simulink model "D_TrigSubsysSin"  (R2019b)
settings: Solver=FixedStepAuto  StartTime=0.0  StopTime=10  FixedStep=0.5  RelTol=1e-3  EnableMultiTasking=on
model workspace (MAT data in the model file):
  AFS = 30
  AS = 0.5
  DT = 5
  cw = 1.3
  g = 9.81
  h0 = 500
  h1 = 150
  m = 85
  rho = 1.2
  v0 = 0
settings Model: Creator=Reichl  LastModifiedBy=jakob
settings DataIOCC: SaveFormat=Array  ReturnWorkspaceOutputs=off  OutputSaveName=h
settings OptimizationCC: LifeSpan=inf
settings DebuggingCC: SolverPrmCheckMsg=warning  SFUnexpectedBacktrackingDiag=warning  SFNoUnconditionalDefaultTransitionDiag=warning  SFExecutionAtInitializationDiag=none  ArithmeticOperatorsInVariantConditions=warning
settings HardwareCC: ProdBitPerPointer=32  ProdBitPerSizeT=32  ProdBitPerPtrDiffT=32  ProdLargestAtomicFloat=None  ProdIntDivRoundTo=Undefined  ProdEndianess=Unspecified  ProdWordSize=32  ProdHWDeviceType=32-bit Generic
settings ModelReferenceCC: PropagateSignalLabelsOutOfModel=off
settings SFSimCC: SimUseLocalCustomCode=off  CustomCodeUndefinedFunction=UseInterfaceOnly
settings RTWCC: RTWUseLocalCustomCode=off
settings CodeAppCC: StateflowObjectComments=on
settings GRTTargetCC: TargetLangStandard=C89/C90 (ANSI)  GeneratePreprocessorConditionals=Disable all
settings ConfigComp: CovMetricSettings=dw  CovHtmlReporting=on  CovSaveCumulativeToWorkspaceVar=on  CovSaveSingleToWorkspaceVar=on  CovExternalEMLEnable=off  CovSFcnEnable=off

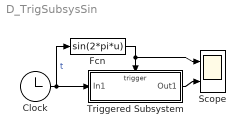
== system D_TrigSubsysSin ==
  Clock : Clock
  Fcn : Fcn  Expr=sin(2*pi*u)
  Scope : Scope  NumInputPorts=2
  Triggered Subsystem : Subsystem  TreatAsAtomicUnit=on
  wires:
  Clock/1 -> Fcn/1, Triggered Subsystem/1(In1)  "t"
  Fcn/1 -> Triggered Subsystem/Trigger, Scope/1
  Triggered Subsystem/1(Out1) -> Scope/2

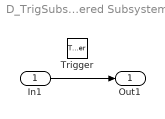
== system D_TrigSubsysSin/Triggered Subsystem ==
  In1 : Inport
  Trigger : TriggerPort  VariantControl=Variant  PortDimensions=1
  Out1 : Outport  SourceOfInitialOutputValue=Input signal  InitialOutput=-0.3  VectorParamsAs1DForOutWhenUnconnected=off
  wires:
  In1/1 -> Out1/1
